simulink model "triac_diac"  (R2018a)
settings: Solver=VariableStepAuto  StartTime=-0.08  StopTime=0.04  MaxStep=1e-6  RelTol=1e-3
libraries: powerlib x35
settings Model: Creator=pdb  LastModifiedBy=pdb
settings DebuggingCC: UnconnectedOutputMsg=none

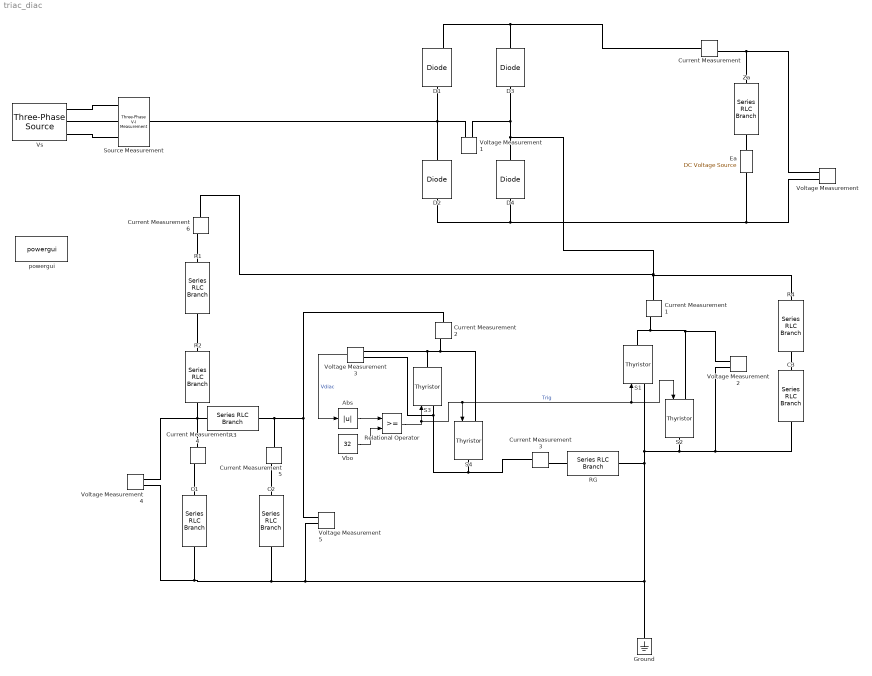
== system triac_diac ==
  Abs : Abs
  C1 : powerlib/Elements/Series RLC Branch  LConnTagsString=__new0  RConnTagsString=__new0  BranchType=C  Resistance=250e3  Inductance=1e-3  SetiL0=off  InitialCurrent=0  Capacitance=0.1e-6  Setx0=off  InitialVoltage=0  Measurements=None
  C2 : powerlib/Elements/Series RLC Branch  LConnTagsString=__new0  RConnTagsString=__new0  BranchType=C  Resistance=250e3  Inductance=1e-3  SetiL0=off  InitialCurrent=0  Capacitance=0.1e-6  Setx0=on  InitialVoltage=10  Measurements=None
  C3 : powerlib/Elements/Series RLC Branch  LConnTagsString=__new0  RConnTagsString=__new0  BranchType=C  Resistance=250e3  Inductance=1e-3  SetiL0=off  InitialCurrent=0  Capacitance=0.1e-6  Setx0=off  InitialVoltage=0  Measurements=None
  Current Measurement{,1..6} (7 alike) : powerlib/Measurements/Current Measurement  PhasorSimulation=off  OutputType=Complex  PSBequivalent=0
  D1 : powerlib/Power Electronics/Diode  Ron=0.01  Lon=0  Vf=1.1  IC=0  UseSnubber=0  Rs=inf  Cs=0  Measurements=on
  D2 : powerlib/Power Electronics/Diode  Ron=0.01  Lon=0  Vf=1.1  IC=0  UseSnubber=0  Rs=inf  Cs=0  Measurements=off
  D3 : powerlib/Power Electronics/Diode  Ron=0.01  Lon=0  Vf=1.1  IC=0  UseSnubber=0  Rs=inf  Cs=0  Measurements=off
  D4 : powerlib/Power Electronics/Diode  Ron=0.01  Lon=0  Vf=1.1  IC=0  UseSnubber=0  Rs=inf  Cs=0  Measurements=off
  Ea : powerlib/Electrical Sources/DC Voltage Source  Amplitude=164  Measurements=None
  Ground : powerlib/Elements/Ground  LConnTagsString=a
  R1 : powerlib/Elements/Series RLC Branch  LConnTagsString=__new0  RConnTagsString=__new0  BranchType=R  Resistance=17e3  Inductance=1e-3  SetiL0=off  InitialCurrent=0  Capacitance=1e-6  Setx0=off  InitialVoltage=0  Measurements=None
  R2 : powerlib/Elements/Series RLC Branch  LConnTagsString=__new0  RConnTagsString=__new0  BranchType=R  Resistance=1e3  Inductance=1e-3  SetiL0=off  InitialCurrent=0  Capacitance=1e-6  Setx0=off  InitialVoltage=0  Measurements=None
  R3 : powerlib/Elements/Series RLC Branch  LConnTagsString=__new0  RConnTagsString=__new0  BranchType=R  Resistance=15e3  Inductance=1e-3  SetiL0=off  InitialCurrent=0  Capacitance=1e-6  Setx0=off  InitialVoltage=0  Measurements=None
  R4 : powerlib/Elements/Series RLC Branch  LConnTagsString=__new0  RConnTagsString=__new0  BranchType=R  Resistance=1000  Inductance=1e-3  SetiL0=off  InitialCurrent=0  Capacitance=1e-6  Setx0=off  InitialVoltage=0  Measurements=None
  RG : powerlib/Elements/Series RLC Branch  LConnTagsString=__new0  RConnTagsString=__new0  BranchType=R  Resistance=300  Inductance=1e-3  SetiL0=off  InitialCurrent=0  Capacitance=1e-6  Setx0=off  InitialVoltage=0  Measurements=None
  Relational Operator : RelationalOperator  OutDataTypeStr=boolean  RndMeth=Simplest
  S1 : powerlib/Power Electronics/Thyristor  Ron=0.016  Lon=0  Vf=1.3  IC=0  Rs=inf  Cs=0  Measurements=off
  S2 : powerlib/Power Electronics/Thyristor  Ron=0.016  Lon=0  Vf=1.3  IC=0  Rs=inf  Cs=0  Measurements=off
  S3 : powerlib/Power Electronics/Thyristor  Ron=0.001  Lon=0  Vf=27  IC=0  Rs=inf  Cs=0  Measurements=off
  S4 : powerlib/Power Electronics/Thyristor  Ron=0.001  Lon=0  Vf=27  IC=0  Rs=inf  Cs=0  Measurements=off
  Source Measurement : powerlib/Measurements/Three-Phase V-I Measurement  VoltageMeasurement=phase-to-ground  SetLabelV=off  LabelV=Vabc  Vpu=off  VpuLL=off  CurrentMeasurement=yes  SetLabelI=off  LabelI=Iabc  Ipu=off  Pbase=100e6  Vbase=500e3  OutputType=Complex  PhasorSimulation=off  PSBequivalent=0
  Vbo : Constant  Value=32
  Voltage Measurement{,1..5} (6 alike) : powerlib/Measurements/Voltage Measurement  PhasorSimulation=off  OutputType=Complex  PSBequivalent=0
  Vs : powerlib/Electrical Sources/Three-Phase Source  InternalConnection=Yg  VoltagePhases=off  Voltage=220*sqrt(3)  PhaseAngle=0  Voltage_phases=[25e3 25e3 25e3]/sqrt(3)  PhaseAngles_phases=[0 -120 +120]  Frequency=50  NonIdealSource=on  SpecifyImpedance=off  Resistance=0.05  Inductance=1.8e-4  ShortCircuitLevel=sqrt(3)*220*20000  BaseVoltage=220*sqrt(3)  XRratio=0.1  BusType=swing  Pref=10e3  Qref=0  Prefabc=[10e3, 10e3, 10e3]  Qrefabc=[0, 0, 0]  Qmin=-inf  Qmax=inf
  Za : powerlib/Elements/Series RLC Branch  LConnTagsString=__new0  RConnTagsString=__new0  BranchType=RL  Resistance=0.8  Inductance=0.0125  SetiL0=off  InitialCurrent=0  Capacitance=1e-6  Setx0=off  InitialVoltage=0  Measurements=None
  powergui : powerlib/powergui  Priority=1  SimulationMode=Continuous  SampleTime=50e-6  frequency=60  Iterations=50  frequencyindice=0  Pbase=100e6  ErrMax=1e-4  UnitsV=kV  UnitsW=MW  buscounter=0  FunctionMessages=off  echomessages=off  EnableUseOfTLC=off  CurrentSourceSwitches=off  DisableSnubberDevices=off  DisableRonSwitches=off  DisableVfSwitches=off  DisplayEquations=off  SolverType=Tustin/Backward Euler (TBE)  Interpol=off  ExternalGateDelay=off  methode=off  Ts=100  x0status=blocks  SPID=on  SwTol=0  HookPort=off  RestoreLinks=warning  ResistiveCurrentMeasurement=off  Frange=[0:2:500]  Ylog=off  Xlog=on  ShowGrid=off  save=off  variable=ZData  structure=0  ZoomFFT=off  StartTime=0.0  cycles=1  DisplayStyle=1  fundamental=60  FreqAxis=off  MaxFrequency=1000  frequencyindicesteady=1  RmsSteady=1  display=off
  wires:
  Relational Operator/1 -> S3/1, S4/1, S1/1, S2/1  "Trig"
  Vbo/1 -> Relational Operator/2
  Abs/1 -> Relational Operator/1
  Voltage Measurement3/1 -> Abs/1  "Vdiac"
  connections:
  Vs/RConn1 -- Source Measurement/LConn1
  Vs/RConn2 -- Source Measurement/LConn2
  Vs/RConn3 -- Source Measurement/LConn3
  Current Measurement/LConn1 -- D1/RConn1 -- D3/RConn1
  Voltage Measurement/LConn2 -- D4/LConn1 -- D2/LConn1 -- Ea/LConn1
  Current Measurement/RConn1 -- Za/LConn1 -- Voltage Measurement/LConn1
  Za/RConn1 -- Ea/RConn1
  C1/RConn1 -- RG/RConn1 -- C3/RConn1 -- Voltage Measurement2/LConn2 -- S2/RConn1 -- S1/LConn1 -- Ground/LConn1 -- Voltage Measurement5/LConn2 -- C2/RConn1 -- Voltage Measurement4/LConn2
  S2/LConn1 -- Voltage Measurement2/LConn1 -- S1/RConn1 -- Current Measurement1/RConn1
  D2/RConn1 -- Voltage Measurement1/LConn1 -- D1/LConn1 -- Source Measurement/RConn1
  D4/RConn1 -- Current Measurement6/LConn1 -- R4/LConn1 -- Current Measurement1/LConn1 -- Voltage Measurement1/LConn2 -- D3/LConn1
  Voltage Measurement3/LConn1 -- S3/RConn1 -- Current Measurement2/RConn1 -- S4/LConn1
  C3/LConn1 -- R4/RConn1
  R3/RConn1 -- Voltage Measurement5/LConn1 -- Current Measurement2/LConn1 -- Current Measurement5/LConn1
  R1/RConn1 -- R2/LConn1
  R2/RConn1 -- Voltage Measurement4/LConn1 -- Current Measurement4/LConn1 -- R3/LConn1
  Current Measurement3/LConn1 -- Voltage Measurement3/LConn2 -- S3/LConn1 -- S4/RConn1
  RG/LConn1 -- Current Measurement3/RConn1
  Current Measurement5/RConn1 -- C2/LConn1
  Current Measurement4/RConn1 -- C1/LConn1
  Current Measurement6/RConn1 -- R1/LConn1
